simulink model "Consumer"  (R2021a)
settings: Solver=VariableStepAuto  StartTime=0.0  StopTime=40  RelTol=1e-3
settings Model: Creator=cm  LastModifiedBy=cm

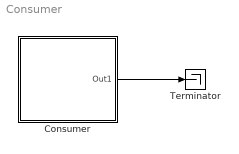
== system Consumer ==
  Consumer : Subsystem
      mask Display: image('250948-200.png'); % Use "Edit Image" on toolstrip to change.
  Terminator : Terminator
  wires:
  Consumer/1(Out1) -> Terminator/1

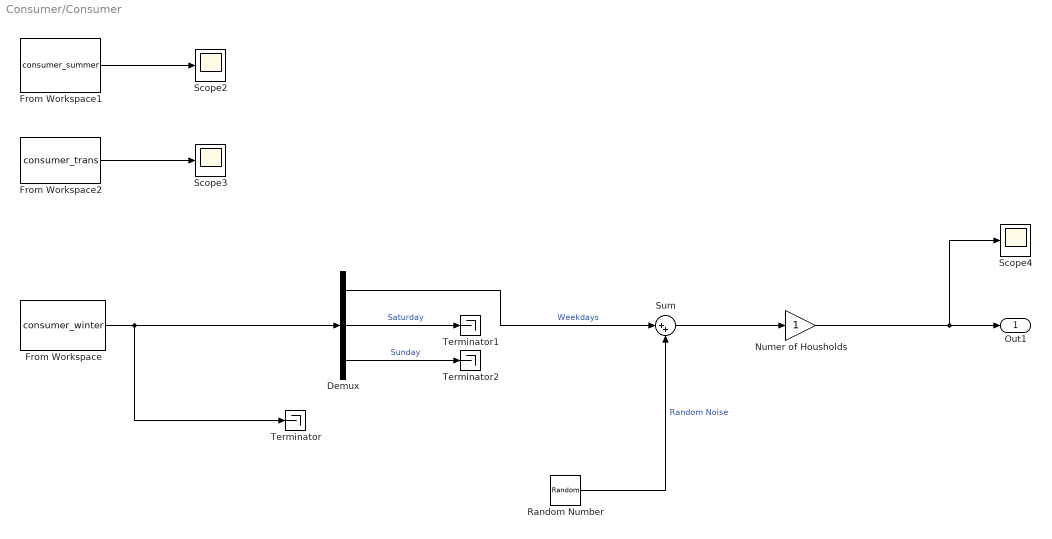
== system Consumer/Consumer ==
  Demux : Demux  Outputs=3
  From Workspace : FromWorkspace  VariableName=consumer_winter  SampleTime=24/96  Interpolate=off  ZeroCross=off  OutputAfterFinalValue=Cyclic repetition
  From Workspace1 : FromWorkspace  VariableName=consumer_summer  SampleTime=24/96  Interpolate=off  ZeroCross=off  OutputAfterFinalValue=Cyclic repetition
  From Workspace2 : FromWorkspace  VariableName=consumer_trans  SampleTime=24/96  Interpolate=off  ZeroCross=off  OutputAfterFinalValue=Cyclic repetition
  Numer of Housholds : Gain
  Random Number : RandomNumber  Variance=0.0001  SampleTime=1
  Scope2 : Scope
  Scope3 : Scope
  Scope4 : Scope
  Sum : Sum  Inputs=|++
  Terminator : Terminator
  Terminator1 : Terminator
  Terminator2 : Terminator
  Out1 : Outport
  wires:
  Demux/2 -> Terminator1/1  "Saturday"
  From Workspace/1 -> Terminator/1, Demux/1
  From Workspace2/1 -> Scope3/1
  Random Number/1 -> Sum/2  "Random Noise"
  Demux/3 -> Terminator2/1  "Sunday"
  Sum/1 -> Numer of Housholds/1
  From Workspace1/1 -> Scope2/1
  Demux/1 -> Sum/1  "Weekdays"
  Numer of Housholds/1 -> Out1/1, Scope4/1
